simulink model "ML"  (Simulink 7.0)
settings: Solver=ode2  StartTime=0.0  StopTime=300  FixedStep=0.1  RelTol=1e-3
values from neighbouring files (symbols this model uses):
  g_K = 36    [executor.m]
undefined symbols (not defined in the file or in its folder): Cm, fai, g_Ca, g_L, V1, V2, V3, V4, V_Ca, V_K, V_L
settings Model: Creator=Administrator  LastModifiedBy=Administrator

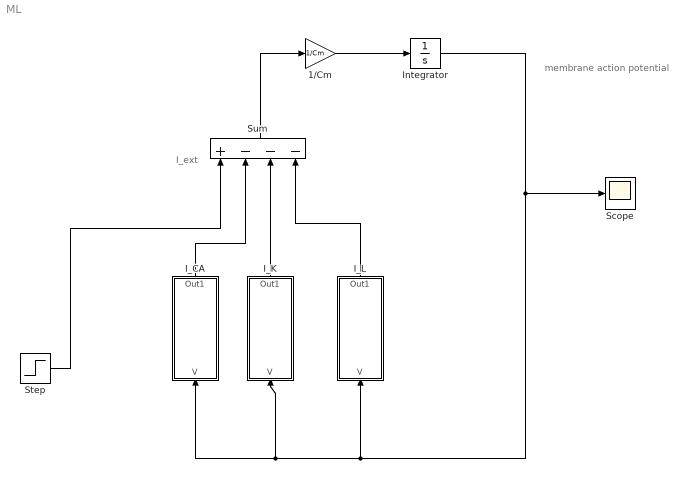
== system ML ==
  note: membrane action potential
  note: I_ext
  1/Cm : Gain  Gain=1/Cm  ParameterDataType=sfix(16)  ParameterScaling=2^0  OutDataType=sfix(16)  OutScaling=2^0
  "I_CA " : Subsystem  Orientation=up
  I_K : Subsystem  Orientation=up
  I_L : Subsystem  Orientation=up
  Integrator : Integrator  InitialCondition=-10
  Scope : Scope
      settings: YMin=-55  YMax=45
  Step : Step  Time=0  After=100  SampleTime=0
  Sum : Sum  Orientation=up  Inputs=+---  OutDataType=sfix(16)  OutScaling=2^0
  wires:
  1/Cm/1 -> Integrator/1
  Integrator/1 -> I_L/1(V), I_K/1(V), "I_CA "/1(V), Scope/1
  Sum/1 -> 1/Cm/1
  I_L/1(Out1) -> Sum/4
  I_K/1(Out1) -> Sum/3
  "I_CA "/1(Out1) -> Sum/2
  Step/1 -> Sum/1

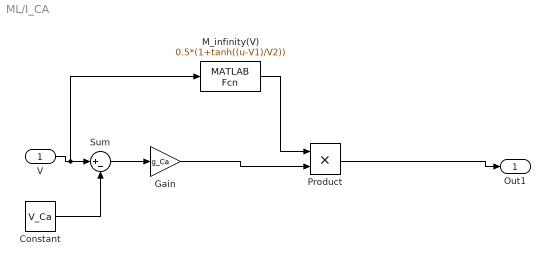
== system ML/I_CA  ==
  V : Inport  OutDataType=sfix(16)  OutScaling=2^0
  Constant : Constant  Value=V_Ca  OutDataType=sfix(16)  OutScaling=2^0
  Gain : Gain  Gain=g_Ca  ParameterDataType=sfix(16)  ParameterScaling=2^0  OutDataType=sfix(16)  OutScaling=2^0
  M_infinity(V) : MATLABFcn  MATLABFcn=0.5*(1+tanh((u-V1)/V2))
  Product : Product  OutDataType=sfix(16)  OutScaling=2^0  RndMeth=Zero
  Sum : Sum  Inputs=|+-  OutDataType=sfix(16)  OutScaling=2^0
  Out1 : Outport  OutDataType=sfix(16)  OutScaling=2^0
  wires:
  V/1 -> Sum/1, M_infinity(V)/1
  Constant/1 -> Sum/2
  Sum/1 -> Gain/1
  Gain/1 -> Product/2
  M_infinity(V)/1 -> Product/1
  Product/1 -> Out1/1

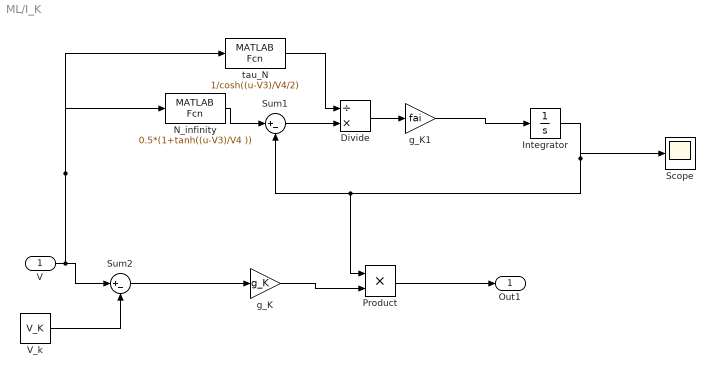
== system ML/I_K ==
  V : Inport  OutDataType=sfix(16)  OutScaling=2^0
  Divide : Product  Inputs=/*  OutDataType=sfix(16)  OutScaling=2^-10
  Integrator : Integrator
  N_infinity : MATLABFcn  MATLABFcn=0.5*(1+tanh((u-V3)/V4 ))
  Product : Product  OutDataType=sfix(16)  OutScaling=2^0  RndMeth=Zero
  Scope : Scope
  Sum1 : Sum  Inputs=|+-  OutDataType=sfix(16)  OutScaling=2^0
  Sum2 : Sum  Inputs=|+-  OutDataType=sfix(16)  OutScaling=2^0
  V_k : Constant  Value=V_K  OutDataType=sfix(16)  OutScaling=2^0
  g_K : Gain  Gain=g_K  ParameterDataType=sfix(16)  ParameterScaling=2^0  OutDataType=sfix(16)  OutScaling=2^0
  g_K1 : Gain  Gain=fai  ParameterDataType=sfix(16)  ParameterScaling=2^0  OutDataType=sfix(16)  OutScaling=2^0
  tau_N : MATLABFcn  MATLABFcn=1/cosh((u-V3)/V4/2)
  Out1 : Outport  OutDataType=sfix(16)  OutScaling=2^0
  wires:
  V/1 -> tau_N/1, N_infinity/1, Sum2/1
  V_k/1 -> Sum2/2
  N_infinity/1 -> Sum1/1
  Integrator/1 -> Sum1/2, Product/1, Scope/1
  tau_N/1 -> Divide/1
  Sum1/1 -> Divide/2
  Divide/1 -> g_K1/1
  g_K1/1 -> Integrator/1
  Sum2/1 -> g_K/1
  g_K/1 -> Product/2
  Product/1 -> Out1/1

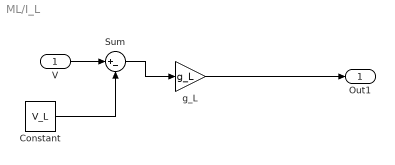
== system ML/I_L ==
  V : Inport  OutDataType=sfix(16)  OutScaling=2^0
  Constant : Constant  Value=V_L  OutDataType=sfix(16)  OutScaling=2^0
  Sum : Sum  Inputs=|+-  OutDataType=sfix(16)  OutScaling=2^0
  g_L : Gain  Gain=g_L  ParameterDataType=sfix(16)  ParameterScaling=2^0  OutDataType=sfix(16)  OutScaling=2^0
  Out1 : Outport  OutDataType=sfix(16)  OutScaling=2^0
  wires:
  V/1 -> Sum/1
  Constant/1 -> Sum/2
  Sum/1 -> g_L/1
  g_L/1 -> Out1/1
